simulink model "tp14"  (R2024b)
settings: Solver=ode23t  StartTime=0.0  StopTime=0.2  FixedStep=0.2  RelTol=1e-4  AbsTol=1e-6  EnableMultiTasking=on
undefined symbols (not defined in the file or in its folder): D1, Delta
libraries: spsThreePhaseVIMeasurementLib x28, spsThreePhaseSeriesRLCBranchLib x20, simulink x14, eePMU x14, spsThreePhaseSeriesRLCLoadLib x11, spsThreePhaseSourceLib x5, spsThreePhaseTransformerTwoWindingsLib x5, spspowerguiLib x1
(part 2 of 2)

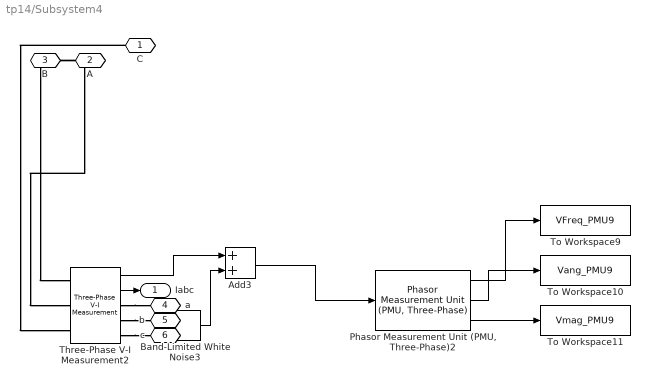
== system tp14/Subsystem4 ==
  Add3 : Sum
  Band-Limited White Noise3 : simulink/Sources/Band-Limited White Noise  Cov=3.16e-8  Ts=0.00833  seed=[23341]
  "Phasor Measurement Unit (PMU, Three-Phase)2" : eePMU/Phasor Measurement Unit (PMU, Three-Phase)  frequency=60  Nsr=64  k=2
      settings: LibrarySourceBlock=|
      | ee_sl_lib/Measurements/Phasor Measurement Unit
      | (PMU, Three-Phase)
  Three-Phase V-I Measurement2 : spsThreePhaseVIMeasurementLib/Three-Phase V-I Measurement  VoltageMeasurement=phase-to-ground  SetLabelV=off  LabelV=Vabc  Vpu=off  VpuLL=off  CurrentMeasurement=yes  SetLabelI=off  LabelI=Iabc  Ipu=off  Pbase=100e6  Vbase=500e3  OutputType=Complex  PhasorSimulation=off  PSBequivalent=0
  To Workspace10 : ToWorkspace  VariableName=Vang_PMU9  SaveFormat=Timeseries  SampleTime=-1
  To Workspace11 : ToWorkspace  VariableName=Vmag_PMU9  SaveFormat=Timeseries  SampleTime=-1
  To Workspace9 : ToWorkspace  VariableName=VFreq_PMU9  SaveFormat=Timeseries  SampleTime=-1
  C : PMIOPort  Side=Left
  A : PMIOPort  Port=2  Side=Left
  B : PMIOPort  Port=3  Side=Left
  a : PMIOPort  Port=4  Side=Right
  b : PMIOPort  Port=5  Side=Right
  c : PMIOPort  Port=6  Side=Right
  Iabc : Outport
  wires:
  "Phasor Measurement Unit (PMU, Three-Phase)2"/1 -> To Workspace9/1
  "Phasor Measurement Unit (PMU, Three-Phase)2"/3 -> To Workspace11/1
  "Phasor Measurement Unit (PMU, Three-Phase)2"/2 -> To Workspace10/1
  Band-Limited White Noise3/1 -> Add3/2
  Add3/1 -> "Phasor Measurement Unit (PMU, Three-Phase)2"/1
  Three-Phase V-I Measurement2/1 -> Add3/1
  Three-Phase V-I Measurement2/2 -> Iabc/1
  connections:
  C/RConn1 -- Three-Phase V-I Measurement2/LConn3
  B/RConn1 -- Three-Phase V-I Measurement2/LConn2
  Three-Phase V-I Measurement2/RConn2 -- b/RConn1
  A/RConn1 -- Three-Phase V-I Measurement2/LConn1
  Three-Phase V-I Measurement2/RConn1 -- a/RConn1
  Three-Phase V-I Measurement2/RConn3 -- c/RConn1

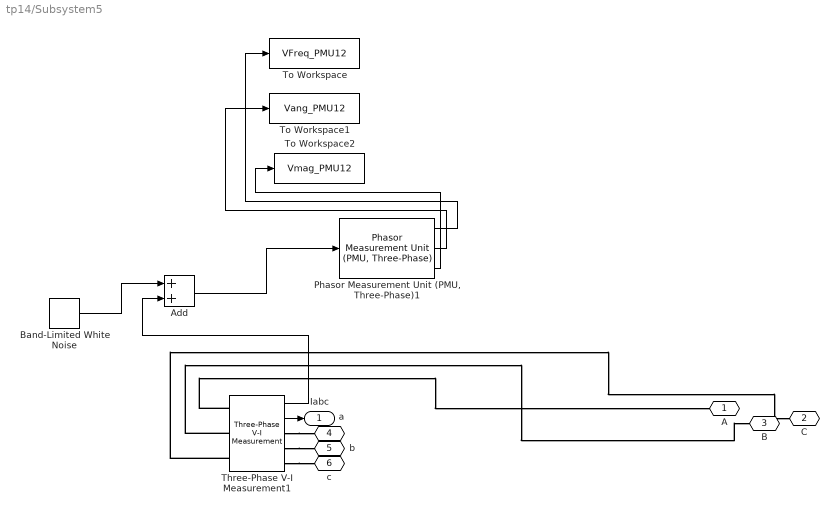
== system tp14/Subsystem5 ==
  Add : Sum
  Band-Limited White Noise : simulink/Sources/Band-Limited White Noise  Cov=3.16e-8  Ts=0.00833  seed=[23341]
  "Phasor Measurement Unit (PMU, Three-Phase)1" : eePMU/Phasor Measurement Unit (PMU, Three-Phase)  frequency=60  Nsr=64  k=2
  Three-Phase V-I Measurement1 : spsThreePhaseVIMeasurementLib/Three-Phase V-I Measurement  VoltageMeasurement=phase-to-ground  SetLabelV=off  LabelV=Vabc  Vpu=off  VpuLL=off  CurrentMeasurement=yes  SetLabelI=off  LabelI=Iabc  Ipu=off  Pbase=100e6  Vbase=500e3  OutputType=Complex  PhasorSimulation=off  PSBequivalent=0
  To Workspace : ToWorkspace  VariableName=VFreq_PMU12  SaveFormat=Timeseries  SampleTime=-1
  To Workspace1 : ToWorkspace  VariableName=Vang_PMU12  SaveFormat=Timeseries  SampleTime=-1
  To Workspace2 : ToWorkspace  VariableName=Vmag_PMU12  SaveFormat=Timeseries  SampleTime=-1
  A : PMIOPort  Side=Left
  C : PMIOPort  Port=2  Side=Left
  B : PMIOPort  Port=3  Side=Left
  a : PMIOPort  Port=4  Side=Right
  b : PMIOPort  Port=5  Side=Right
  c : PMIOPort  Port=6  Side=Right
  Iabc : Outport
  wires:
  Band-Limited White Noise/1 -> Add/1
  "Phasor Measurement Unit (PMU, Three-Phase)1"/2 -> To Workspace1/1
  Three-Phase V-I Measurement1/2 -> Iabc/1
  Add/1 -> "Phasor Measurement Unit (PMU, Three-Phase)1"/1
  "Phasor Measurement Unit (PMU, Three-Phase)1"/1 -> To Workspace/1
  Three-Phase V-I Measurement1/1 -> Add/2
  "Phasor Measurement Unit (PMU, Three-Phase)1"/3 -> To Workspace2/1
  connections:
  Three-Phase V-I Measurement1/LConn2 -- B/RConn1
  Three-Phase V-I Measurement1/RConn3 -- c/RConn1
  Three-Phase V-I Measurement1/RConn1 -- a/RConn1
  Three-Phase V-I Measurement1/RConn2 -- b/RConn1
  Three-Phase V-I Measurement1/LConn3 -- C/RConn1
  Three-Phase V-I Measurement1/LConn1 -- A/RConn1

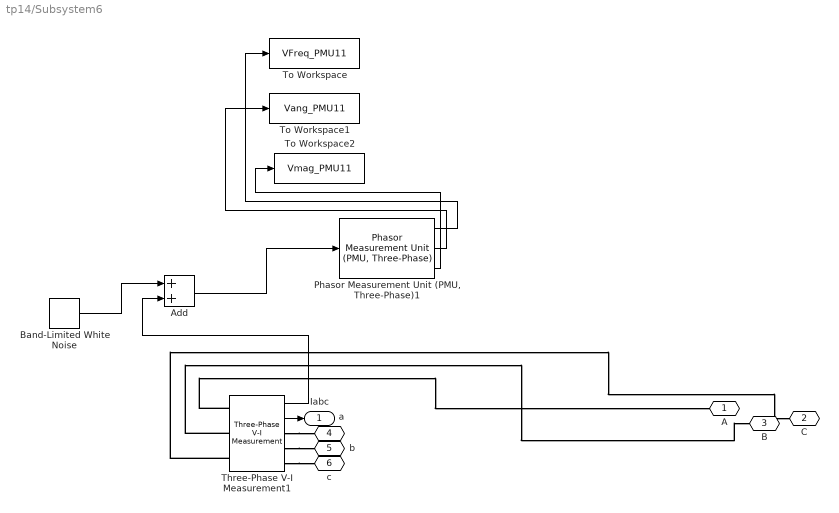
== system tp14/Subsystem6 ==
  Add : Sum
  Band-Limited White Noise : simulink/Sources/Band-Limited White Noise  Cov=3.16e-8  Ts=0.00833  seed=[23341]
  "Phasor Measurement Unit (PMU, Three-Phase)1" : eePMU/Phasor Measurement Unit (PMU, Three-Phase)  frequency=60  Nsr=64  k=2
  Three-Phase V-I Measurement1 : spsThreePhaseVIMeasurementLib/Three-Phase V-I Measurement  VoltageMeasurement=phase-to-ground  SetLabelV=off  LabelV=Vabc  Vpu=off  VpuLL=off  CurrentMeasurement=yes  SetLabelI=off  LabelI=Iabc  Ipu=off  Pbase=100e6  Vbase=500e3  OutputType=Complex  PhasorSimulation=off  PSBequivalent=0
  To Workspace : ToWorkspace  VariableName=VFreq_PMU11  SaveFormat=Timeseries  SampleTime=-1
  To Workspace1 : ToWorkspace  VariableName=Vang_PMU11  SaveFormat=Timeseries  SampleTime=-1
  To Workspace2 : ToWorkspace  VariableName=Vmag_PMU11  SaveFormat=Timeseries  SampleTime=-1
  A : PMIOPort  Side=Left
  C : PMIOPort  Port=2  Side=Left
  B : PMIOPort  Port=3  Side=Left
  a : PMIOPort  Port=4  Side=Right
  b : PMIOPort  Port=5  Side=Right
  c : PMIOPort  Port=6  Side=Right
  Iabc : Outport
  wires:
  Band-Limited White Noise/1 -> Add/1
  "Phasor Measurement Unit (PMU, Three-Phase)1"/2 -> To Workspace1/1
  Three-Phase V-I Measurement1/2 -> Iabc/1
  Add/1 -> "Phasor Measurement Unit (PMU, Three-Phase)1"/1
  "Phasor Measurement Unit (PMU, Three-Phase)1"/1 -> To Workspace/1
  Three-Phase V-I Measurement1/1 -> Add/2
  "Phasor Measurement Unit (PMU, Three-Phase)1"/3 -> To Workspace2/1
  connections:
  Three-Phase V-I Measurement1/LConn2 -- B/RConn1
  Three-Phase V-I Measurement1/RConn3 -- c/RConn1
  Three-Phase V-I Measurement1/RConn1 -- a/RConn1
  Three-Phase V-I Measurement1/RConn2 -- b/RConn1
  Three-Phase V-I Measurement1/LConn3 -- C/RConn1
  Three-Phase V-I Measurement1/LConn1 -- A/RConn1

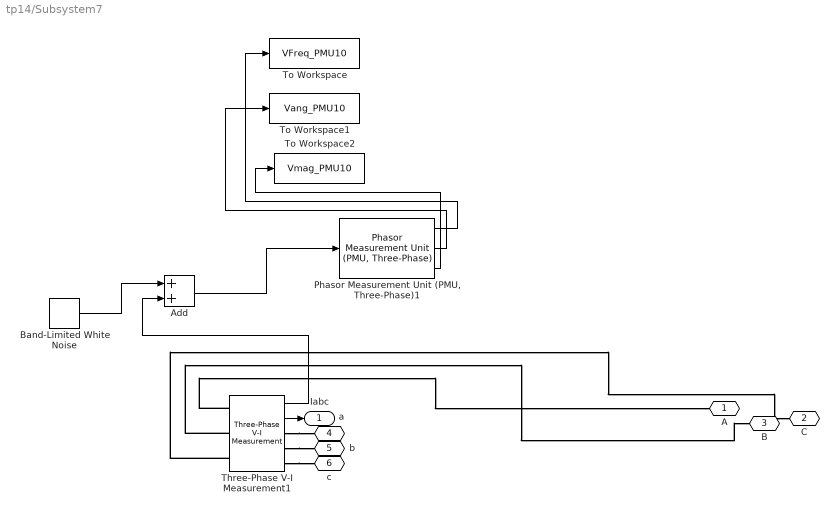
== system tp14/Subsystem7 ==
  Add : Sum
  Band-Limited White Noise : simulink/Sources/Band-Limited White Noise  Cov=3.16e-8  Ts=0.00833  seed=[23341]
  "Phasor Measurement Unit (PMU, Three-Phase)1" : eePMU/Phasor Measurement Unit (PMU, Three-Phase)  frequency=60  Nsr=64  k=2
  Three-Phase V-I Measurement1 : spsThreePhaseVIMeasurementLib/Three-Phase V-I Measurement  VoltageMeasurement=phase-to-ground  SetLabelV=off  LabelV=Vabc  Vpu=off  VpuLL=off  CurrentMeasurement=yes  SetLabelI=off  LabelI=Iabc  Ipu=off  Pbase=100e6  Vbase=500e3  OutputType=Complex  PhasorSimulation=off  PSBequivalent=0
  To Workspace : ToWorkspace  VariableName=VFreq_PMU10  SaveFormat=Timeseries  SampleTime=-1
  To Workspace1 : ToWorkspace  VariableName=Vang_PMU10  SaveFormat=Timeseries  SampleTime=-1
  To Workspace2 : ToWorkspace  VariableName=Vmag_PMU10  SaveFormat=Timeseries  SampleTime=-1
  A : PMIOPort  Side=Left
  C : PMIOPort  Port=2  Side=Left
  B : PMIOPort  Port=3  Side=Left
  a : PMIOPort  Port=4  Side=Right
  b : PMIOPort  Port=5  Side=Right
  c : PMIOPort  Port=6  Side=Right
  Iabc : Outport
  wires:
  Band-Limited White Noise/1 -> Add/1
  "Phasor Measurement Unit (PMU, Three-Phase)1"/2 -> To Workspace1/1
  Three-Phase V-I Measurement1/2 -> Iabc/1
  Add/1 -> "Phasor Measurement Unit (PMU, Three-Phase)1"/1
  "Phasor Measurement Unit (PMU, Three-Phase)1"/1 -> To Workspace/1
  Three-Phase V-I Measurement1/1 -> Add/2
  "Phasor Measurement Unit (PMU, Three-Phase)1"/3 -> To Workspace2/1
  connections:
  Three-Phase V-I Measurement1/LConn2 -- B/RConn1
  Three-Phase V-I Measurement1/RConn3 -- c/RConn1
  Three-Phase V-I Measurement1/RConn1 -- a/RConn1
  Three-Phase V-I Measurement1/RConn2 -- b/RConn1
  Three-Phase V-I Measurement1/LConn3 -- C/RConn1
  Three-Phase V-I Measurement1/LConn1 -- A/RConn1

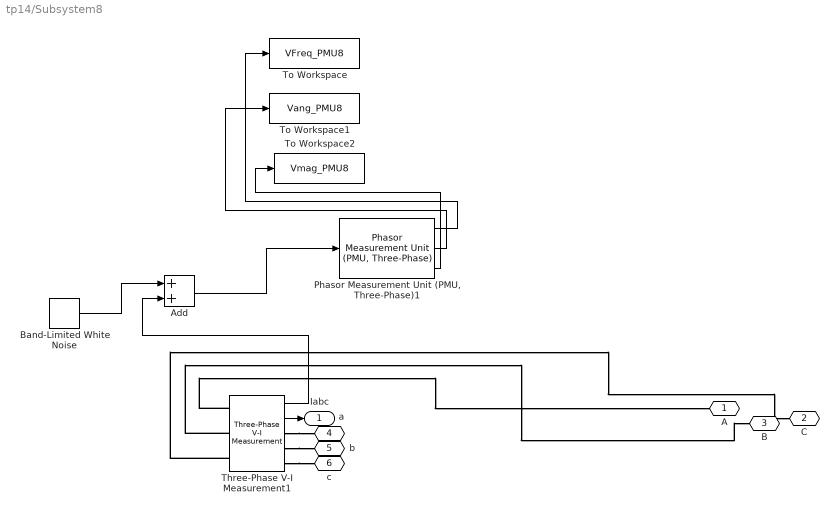
== system tp14/Subsystem8 ==
  Add : Sum
  Band-Limited White Noise : simulink/Sources/Band-Limited White Noise  Cov=3.16e-8  Ts=0.00833  seed=[23341]
  "Phasor Measurement Unit (PMU, Three-Phase)1" : eePMU/Phasor Measurement Unit (PMU, Three-Phase)  frequency=60  Nsr=64  k=2
  Three-Phase V-I Measurement1 : spsThreePhaseVIMeasurementLib/Three-Phase V-I Measurement  VoltageMeasurement=phase-to-ground  SetLabelV=off  LabelV=Vabc  Vpu=off  VpuLL=off  CurrentMeasurement=yes  SetLabelI=off  LabelI=Iabc  Ipu=off  Pbase=100e6  Vbase=500e3  OutputType=Complex  PhasorSimulation=off  PSBequivalent=0
  To Workspace : ToWorkspace  VariableName=VFreq_PMU8  SaveFormat=Timeseries  SampleTime=-1
  To Workspace1 : ToWorkspace  VariableName=Vang_PMU8  SaveFormat=Timeseries  SampleTime=-1
  To Workspace2 : ToWorkspace  VariableName=Vmag_PMU8  SaveFormat=Timeseries  SampleTime=-1
  A : PMIOPort  Side=Left
  C : PMIOPort  Port=2  Side=Left
  B : PMIOPort  Port=3  Side=Left
  a : PMIOPort  Port=4  Side=Right
  b : PMIOPort  Port=5  Side=Right
  c : PMIOPort  Port=6  Side=Right
  Iabc : Outport
  wires:
  Band-Limited White Noise/1 -> Add/1
  "Phasor Measurement Unit (PMU, Three-Phase)1"/2 -> To Workspace1/1
  Three-Phase V-I Measurement1/2 -> Iabc/1
  Add/1 -> "Phasor Measurement Unit (PMU, Three-Phase)1"/1
  "Phasor Measurement Unit (PMU, Three-Phase)1"/1 -> To Workspace/1
  Three-Phase V-I Measurement1/1 -> Add/2
  "Phasor Measurement Unit (PMU, Three-Phase)1"/3 -> To Workspace2/1
  connections:
  Three-Phase V-I Measurement1/LConn2 -- B/RConn1
  Three-Phase V-I Measurement1/RConn3 -- c/RConn1
  Three-Phase V-I Measurement1/RConn1 -- a/RConn1
  Three-Phase V-I Measurement1/RConn2 -- b/RConn1
  Three-Phase V-I Measurement1/LConn3 -- C/RConn1
  Three-Phase V-I Measurement1/LConn1 -- A/RConn1

== system tp14/Subsystem9 ==
  Add : Sum
  Band-Limited White Noise : simulink/Sources/Band-Limited White Noise  Cov=3.16e-8  Ts=0.00833  seed=[23341]
  "Phasor Measurement Unit (PMU, Three-Phase)1" : eePMU/Phasor Measurement Unit (PMU, Three-Phase)  frequency=60  Nsr=64  k=2
  Three-Phase V-I Measurement1 : spsThreePhaseVIMeasurementLib/Three-Phase V-I Measurement  VoltageMeasurement=phase-to-ground  SetLabelV=off  LabelV=Vabc  Vpu=off  VpuLL=off  CurrentMeasurement=yes  SetLabelI=off  LabelI=Iabc  Ipu=off  Pbase=100e6  Vbase=500e3  OutputType=Complex  PhasorSimulation=off  PSBequivalent=0
  To Workspace : ToWorkspace  VariableName=VFreq_PMU3  SaveFormat=Timeseries  SampleTime=-1
  To Workspace1 : ToWorkspace  VariableName=Vang_PMU3  SaveFormat=Timeseries  SampleTime=-1
  To Workspace2 : ToWorkspace  VariableName=Vmag_PMU3  SaveFormat=Timeseries  SampleTime=-1
  A : PMIOPort  Side=Left
  C : PMIOPort  Port=2  Side=Left
  B : PMIOPort  Port=3  Side=Left
  a : PMIOPort  Port=4  Side=Right
  b : PMIOPort  Port=5  Side=Right
  c : PMIOPort  Port=6  Side=Right
  Iabc : Outport
  wires:
  Band-Limited White Noise/1 -> Add/1
  "Phasor Measurement Unit (PMU, Three-Phase)1"/2 -> To Workspace1/1
  Three-Phase V-I Measurement1/2 -> Iabc/1
  Add/1 -> "Phasor Measurement Unit (PMU, Three-Phase)1"/1
  "Phasor Measurement Unit (PMU, Three-Phase)1"/1 -> To Workspace/1
  Three-Phase V-I Measurement1/1 -> Add/2
  "Phasor Measurement Unit (PMU, Three-Phase)1"/3 -> To Workspace2/1
  connections:
  Three-Phase V-I Measurement1/LConn2 -- B/RConn1
  Three-Phase V-I Measurement1/RConn3 -- c/RConn1
  Three-Phase V-I Measurement1/RConn1 -- a/RConn1
  Three-Phase V-I Measurement1/RConn2 -- b/RConn1
  Three-Phase V-I Measurement1/LConn3 -- C/RConn1
  Three-Phase V-I Measurement1/LConn1 -- A/RConn1
